simulink model "cooperative_observer"  (R2024b)
settings: Solver=VariableStepAuto  StartTime=0.0  StopTime=T_sim  RelTol=1e-3
undefined symbols (not defined in the file): A0, Adj, B, C, c, D, F_c, G, K, L0, noise_level, noise_sample_time, x0_0, x0_1, x0_2, x0_3, x0_4, x0_5, x0_6, x0_hat
libraries: simulink x7
settings Model: Creator=fvero  LastModifiedBy=fvero

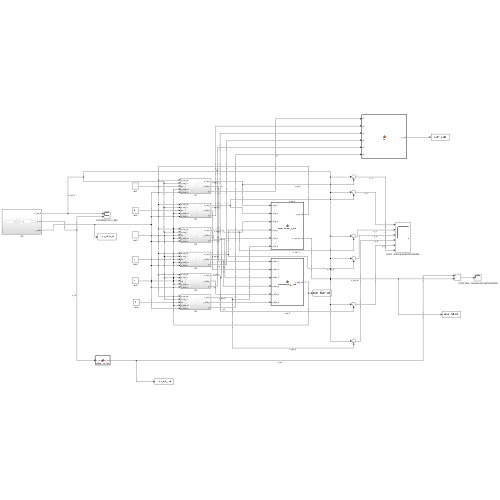
[thumbnail: Simulink's stored preview of the top-level diagram]
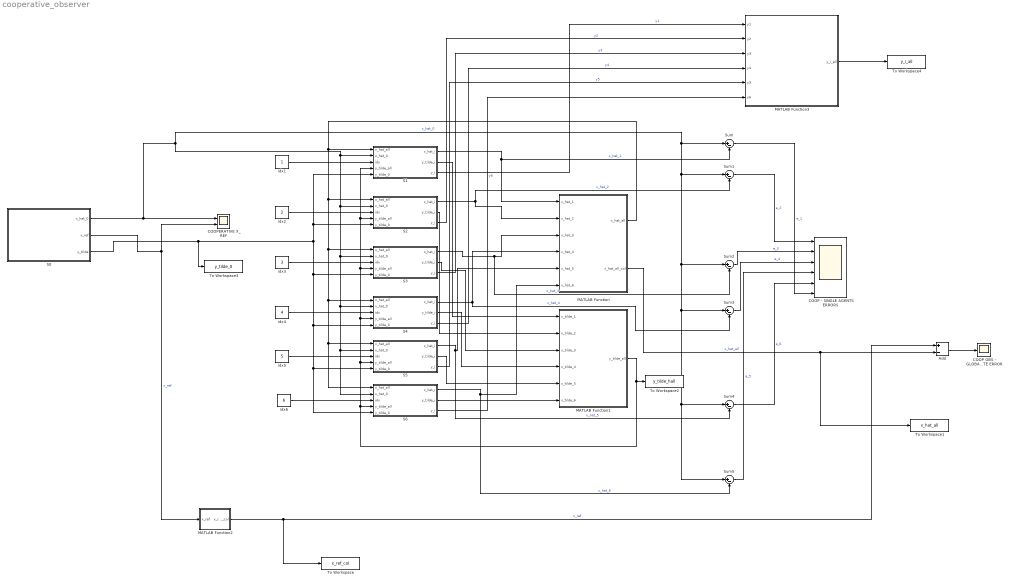
== system cooperative_observer ==
  Add : Sum  Inputs=+-
  "COOP - SINGLE AGENTS ERRORS " : Scope  NumInputPorts=6
  COOP OBS - GLOBAL ESTIMATE ERROR : Scope
  COOPERATIVE X_REF : Scope  NumInputPorts=2
  MATLAB Function : MATLAB Function  TreatAsAtomicUnit=on
  MATLAB Function1 : MATLAB Function  TreatAsAtomicUnit=on
  MATLAB Function2 : MATLAB Function  TreatAsAtomicUnit=on
  MATLAB Function3 : MATLAB Function  TreatAsAtomicUnit=on
  S0 : Subsystem
  S1 : Subsystem
  S2 : Subsystem
  S3 : Subsystem
  S4 : Subsystem
  S5 : Subsystem
  S6 : Subsystem
  Sum{,1..5} (6 alike) : Sum  Inputs=|+-
  To Workspace : ToWorkspace  VariableName=x_ref_col  SaveFormat=Timeseries  SampleTime=-1
  To Workspace1 : ToWorkspace  VariableName=x_hat_all  SaveFormat=Timeseries  SampleTime=-1
  To Workspace2 : ToWorkspace  VariableName=y_tilde_hall  SaveFormat=Timeseries  SampleTime=-1
  To Workspace3 : ToWorkspace  VariableName=y_tilde_0  SaveFormat=Timeseries  SampleTime=-1
  To Workspace4 : ToWorkspace  VariableName=y_i_all  SaveFormat=Timeseries  SampleTime=-1
  idx1 : Constant
  idx2 : Constant  Value=2
  idx3 : Constant  Value=3
  idx4 : Constant  Value=4
  idx5 : Constant  Value=5
  idx6 : Constant  Value=6
  wires:
  MATLAB Function/1(x_hat_all) -> S2/1(x_hat_all), S3/1(x_hat_all), S6/1(x_hat_all), S5/1(x_hat_all), S4/1(x_hat_all), S1/1(x_hat_all)
  idx1/1 -> S1/3(idx)
  idx2/1 -> S2/3(idx)
  idx3/1 -> S3/3(idx)
  idx4/1 -> S4/3(idx)
  idx6/1 -> S6/3(idx)
  idx5/1 -> S5/3(idx)
  S0/1(x_hat_0) -> S2/2(x_hat_0), S3/2(x_hat_0), S6/2(x_hat_0), S5/2(x_hat_0), S4/2(x_hat_0), S1/2(x_hat_0), Sum4/1, Sum5/1, Sum3/1, Sum2/1, Sum1/1, Sum/1, COOPERATIVE X_REF/1  "x_hat_0"
  S1/1(x_hat_i) -> Sum/2, MATLAB Function/1(x_hat_1)  "x_hat_1"
  S2/1(x_hat_i) -> MATLAB Function/2(x_hat_2), Sum1/2  "x_hat_2"
  S3/1(x_hat_i) -> Sum2/2, MATLAB Function/3(x_hat_3)  "x_hat_3"
  S4/1(x_hat_i) -> MATLAB Function/4(x_hat_4), Sum3/2  "x_hat_4"
  S5/1(x_hat_i) -> Sum4/2, MATLAB Function/5(x_hat_5)  "x_hat_5"
  S6/1(x_hat_i) -> Sum5/2, MATLAB Function/6(x_hat_6)  "x_hat_6"
  S1/2(y_tilde_i) -> MATLAB Function1/1(x_tilde_1)
  S2/2(y_tilde_i) -> MATLAB Function1/2(x_tilde_2)
  S3/2(y_tilde_i) -> MATLAB Function1/3(x_tilde_3)
  S4/2(y_tilde_i) -> MATLAB Function1/4(x_tilde_4)
  S5/2(y_tilde_i) -> MATLAB Function1/5(x_tilde_5)
  S6/2(y_tilde_i) -> MATLAB Function1/6(x_tilde_6)
  MATLAB Function1/1(y_tilde_all) -> To Workspace2/1, S6/4(y_tilde_all), S5/4(y_tilde_all), S4/4(y_tilde_all), S3/4(y_tilde_all), S2/4(y_tilde_all), S1/4(y_tilde_all)
  S0/3(y_tilde) -> To Workspace3/1, S2/5(y_tilde_0), S1/5(y_tilde_0), S3/5(y_tilde_0), S6/5(y_tilde_0), S5/5(y_tilde_0), S4/5(y_tilde_0)
  MATLAB Function/2(x_hat_all_col) -> To Workspace1/1, Add/2  "x_hat_all"
  S0/2(x_ref) -> MATLAB Function2/1(x_ref), COOPERATIVE X_REF/2  "x_ref"
  MATLAB Function2/1(x_ref_col) -> To Workspace/1, Add/1  "x_ref"
  Add/1 -> COOP OBS - GLOBAL ESTIMATE ERROR/1
  Sum/1 -> "COOP - SINGLE AGENTS ERRORS "/6  "e_1"
  Sum1/1 -> "COOP - SINGLE AGENTS ERRORS "/1  "e_2"
  Sum2/1 -> "COOP - SINGLE AGENTS ERRORS "/2  "e_3"
  Sum3/1 -> "COOP - SINGLE AGENTS ERRORS "/3  "e_4"
  Sum4/1 -> "COOP - SINGLE AGENTS ERRORS "/5  "e_6"
  Sum5/1 -> "COOP - SINGLE AGENTS ERRORS "/4  "e_5"
  S1/3(y_i) -> MATLAB Function3/1(y1)  "y1"
  S2/3(y_i) -> MATLAB Function3/2(y2)  "y2"
  S3/3(y_i) -> MATLAB Function3/3(y3)  "y3"
  S4/3(y_i) -> MATLAB Function3/4(y4)  "y4"
  S5/3(y_i) -> MATLAB Function3/5(y5)  "y5"
  S6/3(y_i) -> MATLAB Function3/6(y6)  "y6"
  MATLAB Function3/1(y_i_all) -> To Workspace4/1

== system cooperative_observer/S0 ==
  Leader Observer : Subsystem
  Subsystem : Subsystem
  To Workspace : ToWorkspace  VariableName=y_ref  SaveFormat=Timeseries  SampleTime=-1
  x_hat_0 : Outport
  x_ref : Outport  Port=2
  y_tilde : Outport  Port=3
  wires:
  Subsystem/1(y_ref) -> To Workspace/1, Leader Observer/1(y)
  Leader Observer/1(x_hat_0) -> x_hat_0/1
  Subsystem/2(x_ref) -> x_ref/1
  Leader Observer/2(y_tilde) -> y_tilde/1

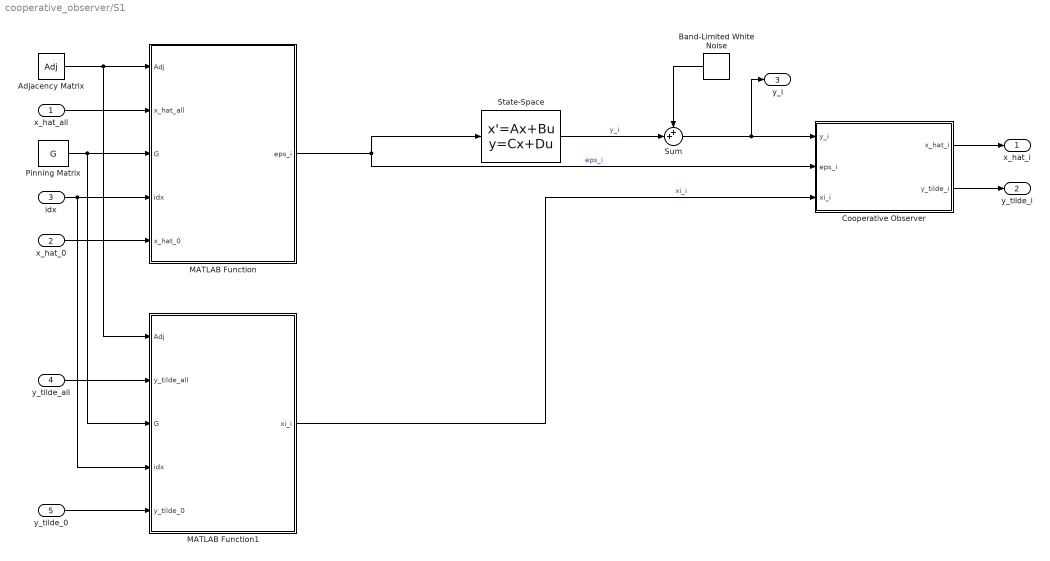
== system cooperative_observer/S1 ==
  x_hat_all : Inport
  x_hat_0 : Inport  Port=2
  idx : Inport  Port=3
  y_tilde_all : Inport  Port=4
  y_tilde_0 : Inport  Port=5
  "Adjacency Matrix " : Constant  Value=Adj
  Band-Limited White Noise : simulink/Sources/Band-Limited White Noise  Cov=[noise_level]  Ts=noise_sample_time  seed=[42]
  Cooperative Observer : Subsystem
  MATLAB Function : MATLAB Function  TreatAsAtomicUnit=on
  MATLAB Function1 : MATLAB Function  TreatAsAtomicUnit=on
  Pinning Matrix : Constant  Value=G
  State-Space : StateSpace  A=A0  B=c*B*K  C=C  D=D  InitialCondition=x0_1
  Sum : Sum  Inputs=++|
  x_hat_i : Outport
  y_tilde_i : Outport  Port=2
  y_i : Outport  Port=3
  wires:
  MATLAB Function/1(eps_i) -> State-Space/1, Cooperative Observer/2(eps_i)  "eps_i"
  x_hat_all/1 -> MATLAB Function/2(x_hat_all)
  x_hat_0/1 -> MATLAB Function/5(x_hat_0)
  Pinning Matrix/1 -> MATLAB Function1/3(G), MATLAB Function/3(G)
  "Adjacency Matrix "/1 -> MATLAB Function1/1(Adj), MATLAB Function/1(Adj)
  idx/1 -> MATLAB Function1/4(idx), MATLAB Function/4(idx)
  Cooperative Observer/1(x_hat_i) -> x_hat_i/1
  Cooperative Observer/2(y_tilde_i) -> y_tilde_i/1
  y_tilde_all/1 -> MATLAB Function1/2(y_tilde_all)
  y_tilde_0/1 -> MATLAB Function1/5(y_tilde_0)
  MATLAB Function1/1(xi_i) -> Cooperative Observer/3(xi_i)  "xi_i"
  Band-Limited White Noise/1 -> Sum/1
  State-Space/1 -> Sum/2  "y_i"
  Sum/1 -> y_i/1, Cooperative Observer/1(y_i)

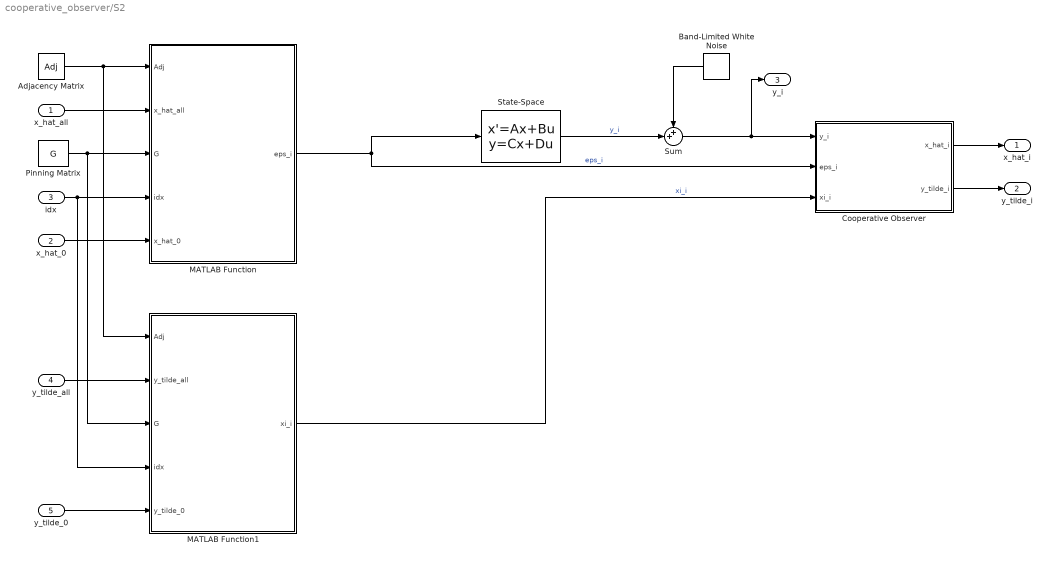
== system cooperative_observer/S2 ==
  x_hat_all : Inport
  x_hat_0 : Inport  Port=2
  idx : Inport  Port=3
  y_tilde_all : Inport  Port=4
  y_tilde_0 : Inport  Port=5
  "Adjacency Matrix " : Constant  Value=Adj
  Band-Limited White Noise : simulink/Sources/Band-Limited White Noise  Cov=[noise_level]  Ts=noise_sample_time  seed=[42]
  Cooperative Observer : Subsystem
  MATLAB Function : MATLAB Function  TreatAsAtomicUnit=on
  MATLAB Function1 : MATLAB Function  TreatAsAtomicUnit=on
  Pinning Matrix : Constant  Value=G
  State-Space : StateSpace  A=A0  B=c*B*K  C=C  D=D  InitialCondition=x0_2
  Sum : Sum  Inputs=++|
  x_hat_i : Outport
  y_tilde_i : Outport  Port=2
  y_i : Outport  Port=3
  wires:
  MATLAB Function/1(eps_i) -> State-Space/1, Cooperative Observer/2(eps_i)  "eps_i"
  x_hat_all/1 -> MATLAB Function/2(x_hat_all)
  x_hat_0/1 -> MATLAB Function/5(x_hat_0)
  Pinning Matrix/1 -> MATLAB Function1/3(G), MATLAB Function/3(G)
  "Adjacency Matrix "/1 -> MATLAB Function1/1(Adj), MATLAB Function/1(Adj)
  idx/1 -> MATLAB Function1/4(idx), MATLAB Function/4(idx)
  Cooperative Observer/1(x_hat_i) -> x_hat_i/1
  Cooperative Observer/2(y_tilde_i) -> y_tilde_i/1
  y_tilde_all/1 -> MATLAB Function1/2(y_tilde_all)
  y_tilde_0/1 -> MATLAB Function1/5(y_tilde_0)
  MATLAB Function1/1(xi_i) -> Cooperative Observer/3(xi_i)  "xi_i"
  Band-Limited White Noise/1 -> Sum/1
  State-Space/1 -> Sum/2  "y_i"
  Sum/1 -> y_i/1, Cooperative Observer/1(y_i)

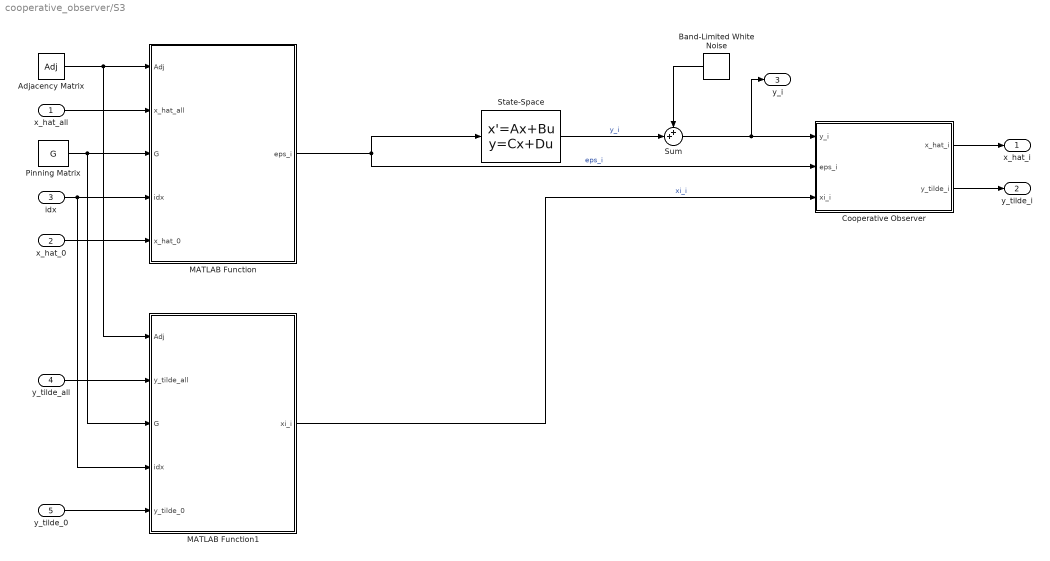
== system cooperative_observer/S3 ==
  x_hat_all : Inport
  x_hat_0 : Inport  Port=2
  idx : Inport  Port=3
  y_tilde_all : Inport  Port=4
  y_tilde_0 : Inport  Port=5
  "Adjacency Matrix " : Constant  Value=Adj
  Band-Limited White Noise : simulink/Sources/Band-Limited White Noise  Cov=[noise_level]  Ts=noise_sample_time  seed=[42]
  Cooperative Observer : Subsystem
  MATLAB Function : MATLAB Function  TreatAsAtomicUnit=on
  MATLAB Function1 : MATLAB Function  TreatAsAtomicUnit=on
  Pinning Matrix : Constant  Value=G
  State-Space : StateSpace  A=A0  B=c*B*K  C=C  D=D  InitialCondition=x0_3
  Sum : Sum  Inputs=++|
  x_hat_i : Outport
  y_tilde_i : Outport  Port=2
  y_i : Outport  Port=3
  wires:
  MATLAB Function/1(eps_i) -> State-Space/1, Cooperative Observer/2(eps_i)  "eps_i"
  x_hat_all/1 -> MATLAB Function/2(x_hat_all)
  x_hat_0/1 -> MATLAB Function/5(x_hat_0)
  Pinning Matrix/1 -> MATLAB Function1/3(G), MATLAB Function/3(G)
  "Adjacency Matrix "/1 -> MATLAB Function1/1(Adj), MATLAB Function/1(Adj)
  idx/1 -> MATLAB Function1/4(idx), MATLAB Function/4(idx)
  Cooperative Observer/1(x_hat_i) -> x_hat_i/1
  Cooperative Observer/2(y_tilde_i) -> y_tilde_i/1
  y_tilde_all/1 -> MATLAB Function1/2(y_tilde_all)
  y_tilde_0/1 -> MATLAB Function1/5(y_tilde_0)
  MATLAB Function1/1(xi_i) -> Cooperative Observer/3(xi_i)  "xi_i"
  Band-Limited White Noise/1 -> Sum/1
  State-Space/1 -> Sum/2  "y_i"
  Sum/1 -> y_i/1, Cooperative Observer/1(y_i)

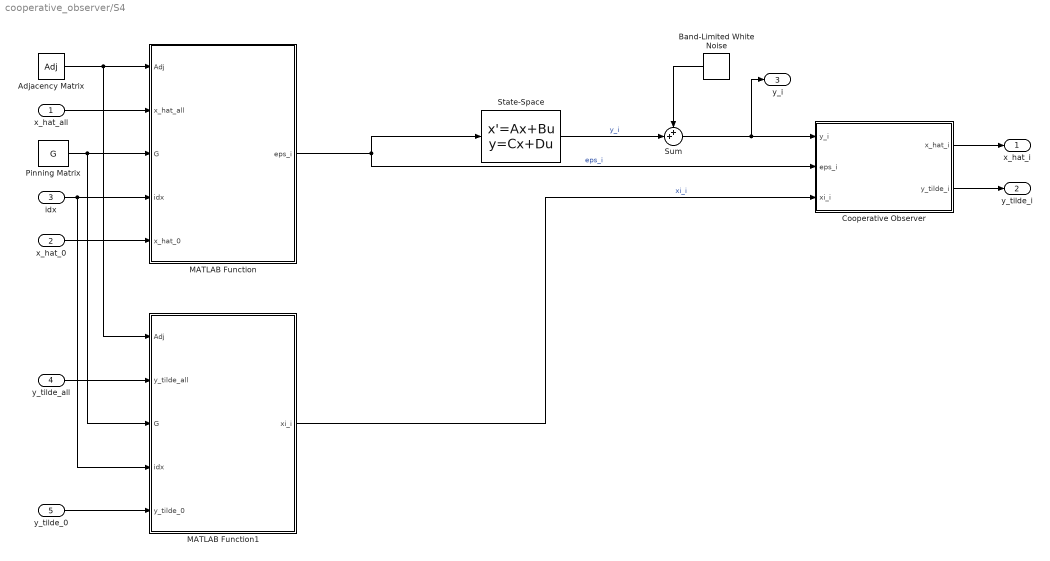
== system cooperative_observer/S4 ==
  x_hat_all : Inport
  x_hat_0 : Inport  Port=2
  idx : Inport  Port=3
  y_tilde_all : Inport  Port=4
  y_tilde_0 : Inport  Port=5
  "Adjacency Matrix " : Constant  Value=Adj
  Band-Limited White Noise : simulink/Sources/Band-Limited White Noise  Cov=[noise_level]  Ts=noise_sample_time  seed=[42]
  Cooperative Observer : Subsystem
  MATLAB Function : MATLAB Function  TreatAsAtomicUnit=on
  MATLAB Function1 : MATLAB Function  TreatAsAtomicUnit=on
  Pinning Matrix : Constant  Value=G
  State-Space : StateSpace  A=A0  B=c*B*K  C=C  D=D  InitialCondition=x0_4
  Sum : Sum  Inputs=++|
  x_hat_i : Outport
  y_tilde_i : Outport  Port=2
  y_i : Outport  Port=3
  wires:
  MATLAB Function/1(eps_i) -> State-Space/1, Cooperative Observer/2(eps_i)  "eps_i"
  x_hat_all/1 -> MATLAB Function/2(x_hat_all)
  x_hat_0/1 -> MATLAB Function/5(x_hat_0)
  Pinning Matrix/1 -> MATLAB Function1/3(G), MATLAB Function/3(G)
  "Adjacency Matrix "/1 -> MATLAB Function1/1(Adj), MATLAB Function/1(Adj)
  idx/1 -> MATLAB Function1/4(idx), MATLAB Function/4(idx)
  Cooperative Observer/1(x_hat_i) -> x_hat_i/1
  Cooperative Observer/2(y_tilde_i) -> y_tilde_i/1
  y_tilde_all/1 -> MATLAB Function1/2(y_tilde_all)
  y_tilde_0/1 -> MATLAB Function1/5(y_tilde_0)
  MATLAB Function1/1(xi_i) -> Cooperative Observer/3(xi_i)  "xi_i"
  Band-Limited White Noise/1 -> Sum/1
  State-Space/1 -> Sum/2  "y_i"
  Sum/1 -> y_i/1, Cooperative Observer/1(y_i)

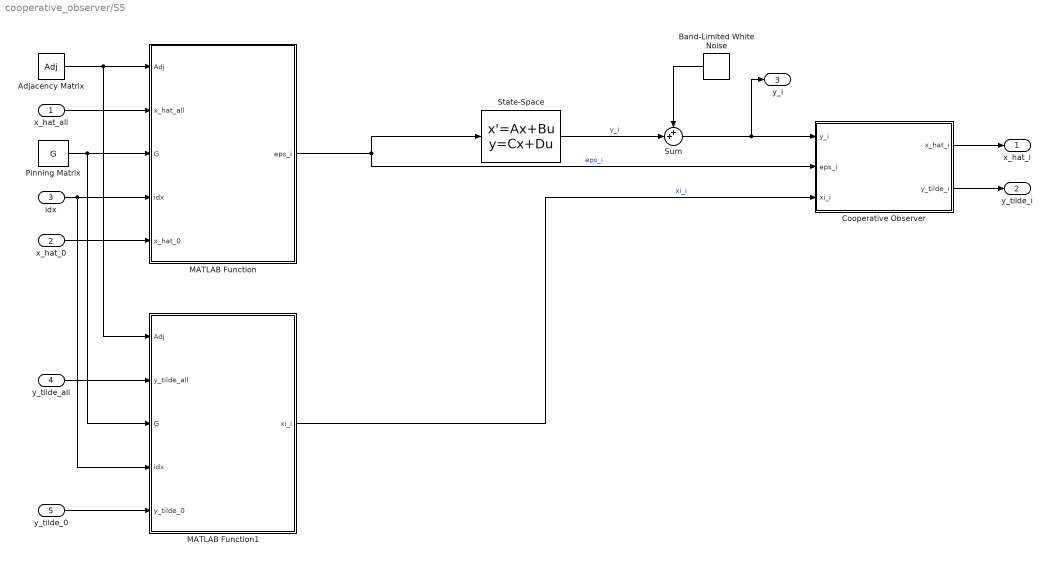
== system cooperative_observer/S5 ==
  x_hat_all : Inport
  x_hat_0 : Inport  Port=2
  idx : Inport  Port=3
  y_tilde_all : Inport  Port=4
  y_tilde_0 : Inport  Port=5
  "Adjacency Matrix " : Constant  Value=Adj
  Band-Limited White Noise : simulink/Sources/Band-Limited White Noise  Cov=[noise_level]  Ts=noise_sample_time  seed=[42]
  Cooperative Observer : Subsystem
  MATLAB Function : MATLAB Function  TreatAsAtomicUnit=on
  MATLAB Function1 : MATLAB Function  TreatAsAtomicUnit=on
  Pinning Matrix : Constant  Value=G
  State-Space : StateSpace  A=A0  B=c*B*K  C=C  D=D  InitialCondition=x0_5
  Sum : Sum  Inputs=++|
  x_hat_i : Outport
  y_tilde_i : Outport  Port=2
  y_i : Outport  Port=3
  wires:
  MATLAB Function/1(eps_i) -> State-Space/1, Cooperative Observer/2(eps_i)  "eps_i"
  x_hat_all/1 -> MATLAB Function/2(x_hat_all)
  x_hat_0/1 -> MATLAB Function/5(x_hat_0)
  Pinning Matrix/1 -> MATLAB Function1/3(G), MATLAB Function/3(G)
  "Adjacency Matrix "/1 -> MATLAB Function1/1(Adj), MATLAB Function/1(Adj)
  idx/1 -> MATLAB Function1/4(idx), MATLAB Function/4(idx)
  Cooperative Observer/1(x_hat_i) -> x_hat_i/1
  Cooperative Observer/2(y_tilde_i) -> y_tilde_i/1
  y_tilde_all/1 -> MATLAB Function1/2(y_tilde_all)
  y_tilde_0/1 -> MATLAB Function1/5(y_tilde_0)
  MATLAB Function1/1(xi_i) -> Cooperative Observer/3(xi_i)  "xi_i"
  Band-Limited White Noise/1 -> Sum/1
  State-Space/1 -> Sum/2  "y_i"
  Sum/1 -> y_i/1, Cooperative Observer/1(y_i)

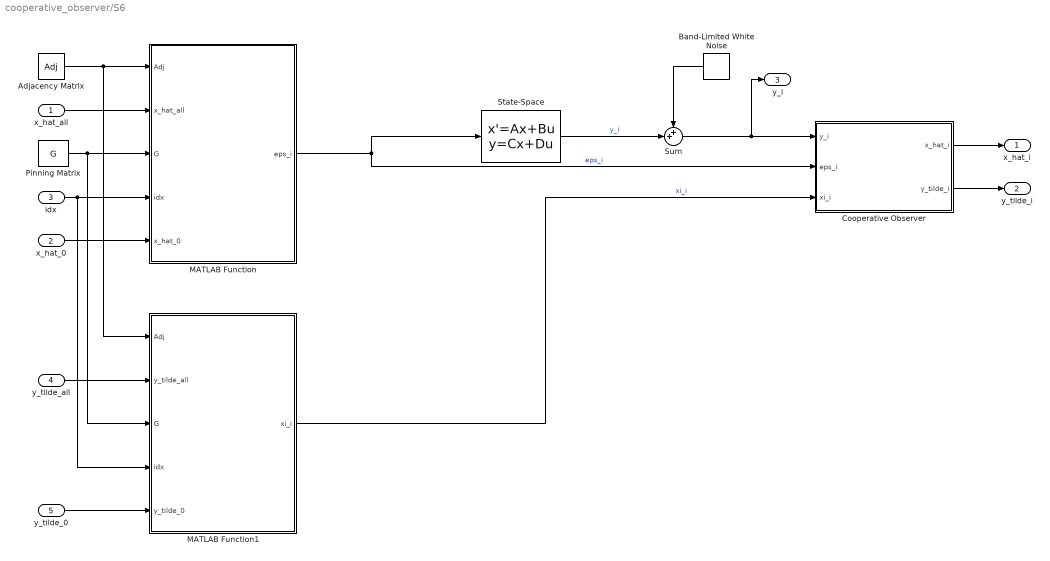
== system cooperative_observer/S6 ==
  x_hat_all : Inport
  x_hat_0 : Inport  Port=2
  idx : Inport  Port=3
  y_tilde_all : Inport  Port=4
  y_tilde_0 : Inport  Port=5
  "Adjacency Matrix " : Constant  Value=Adj
  Band-Limited White Noise : simulink/Sources/Band-Limited White Noise  Cov=[noise_level]  Ts=noise_sample_time  seed=[42]
  Cooperative Observer : Subsystem
  MATLAB Function : MATLAB Function  TreatAsAtomicUnit=on
  MATLAB Function1 : MATLAB Function  TreatAsAtomicUnit=on
  Pinning Matrix : Constant  Value=G
  State-Space : StateSpace  A=A0  B=c*B*K  C=C  D=D  InitialCondition=x0_6
  Sum : Sum  Inputs=++|
  x_hat_i : Outport
  y_tilde_i : Outport  Port=2
  y_i : Outport  Port=3
  wires:
  MATLAB Function/1(eps_i) -> State-Space/1, Cooperative Observer/2(eps_i)  "eps_i"
  x_hat_all/1 -> MATLAB Function/2(x_hat_all)
  x_hat_0/1 -> MATLAB Function/5(x_hat_0)
  Pinning Matrix/1 -> MATLAB Function1/3(G), MATLAB Function/3(G)
  "Adjacency Matrix "/1 -> MATLAB Function1/1(Adj), MATLAB Function/1(Adj)
  idx/1 -> MATLAB Function1/4(idx), MATLAB Function/4(idx)
  Cooperative Observer/1(x_hat_i) -> x_hat_i/1
  Cooperative Observer/2(y_tilde_i) -> y_tilde_i/1
  y_tilde_all/1 -> MATLAB Function1/2(y_tilde_all)
  y_tilde_0/1 -> MATLAB Function1/5(y_tilde_0)
  MATLAB Function1/1(xi_i) -> Cooperative Observer/3(xi_i)  "xi_i"
  Band-Limited White Noise/1 -> Sum/1
  State-Space/1 -> Sum/2  "y_i"
  Sum/1 -> y_i/1, Cooperative Observer/1(y_i)

== system cooperative_observer/S0/Leader Observer ==
  y : Inport
  Add : Sum
  Add1 : Sum  Inputs=+-
  Band-Limited White Noise : simulink/Sources/Band-Limited White Noise  Cov=noise_level  Ts=noise_sample_time  seed=[42]
  Gain1 : Gain  Gain=A0  Multiplication=Matrix(K*u)
  Gain2 : Gain  Gain=C  Multiplication=Matrix(K*u)
  Gain3 : Gain  Gain=c*L0  Multiplication=Matrix(K*u)
  Integrator : Integrator  InitialCondition=[0, 0]'
  Sum : Sum  Inputs=|++
  x_hat_0 : Outport
  y_tilde : Outport  Port=2
  wires:
  Add/1 -> Integrator/1  "x_hat_dot"
  Integrator/1 -> x_hat_0/1, Gain2/1, Gain1/1  "x_hat"
  Gain2/1 -> Add1/2  "y_hat"
  Gain1/1 -> Add/2
  Add1/1 -> y_tilde/1, Gain3/1  "y_tilde"
  Gain3/1 -> Add/1
  Band-Limited White Noise/1 -> Sum/2
  y/1 -> Sum/1
  Sum/1 -> Add1/1

== system cooperative_observer/S0/Subsystem ==
  Gain : Gain  Gain=C  Multiplication=Matrix(K*u)
  Gain1 : Gain  Gain=A0  Multiplication=Matrix(K*u)
  Integrator : Integrator  InitialCondition=x0_0
  y_ref : Outport
  x_ref : Outport  Port=2
  wires:
  Gain1/1 -> Integrator/1
  Integrator/1 -> Gain1/1, Gain/1, x_ref/1
  Gain/1 -> y_ref/1

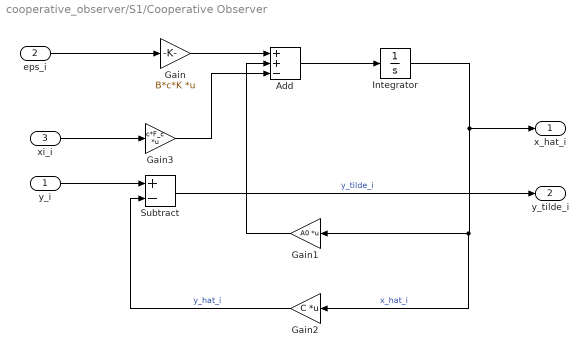
== system cooperative_observer/S1/Cooperative Observer ==
  y_i : Inport
  eps_i : Inport  Port=2
  xi_i : Inport  Port=3
  Add : Sum  Inputs=++-
  Gain : Gain  Gain=B*c*K  Multiplication=Matrix(K*u)
  Gain1 : Gain  Gain=A0  Multiplication=Matrix(K*u)
  Gain2 : Gain  Gain=C  Multiplication=Matrix(K*u)
  Gain3 : Gain  Gain=c*F_c  Multiplication=Matrix(K*u)
  Integrator : Integrator  InitialCondition=x0_hat
  Subtract : Sum  Inputs=+-
  x_hat_i : Outport
  y_tilde_i : Outport  Port=2
  wires:
  eps_i/1 -> Gain/1
  Integrator/1 -> Gain2/1, Gain1/1, x_hat_i/1  "x_hat_i"
  y_i/1 -> Subtract/1
  Gain2/1 -> Subtract/2  "y_hat_i"
  Subtract/1 -> y_tilde_i/1  "y_tilde_i"
  Gain/1 -> Add/1
  Gain3/1 -> Add/3
  Gain1/1 -> Add/2
  Add/1 -> Integrator/1
  xi_i/1 -> Gain3/1

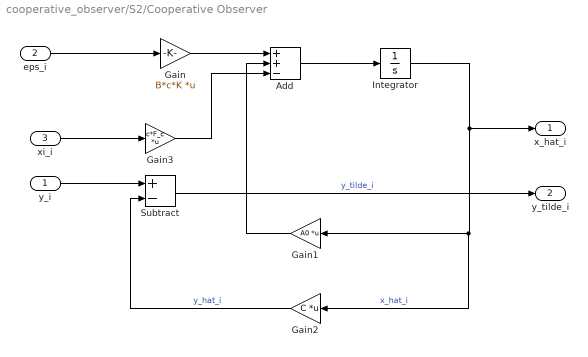
== system cooperative_observer/S2/Cooperative Observer ==
  y_i : Inport
  eps_i : Inport  Port=2
  xi_i : Inport  Port=3
  Add : Sum  Inputs=++-
  Gain : Gain  Gain=B*c*K  Multiplication=Matrix(K*u)
  Gain1 : Gain  Gain=A0  Multiplication=Matrix(K*u)
  Gain2 : Gain  Gain=C  Multiplication=Matrix(K*u)
  Gain3 : Gain  Gain=c*F_c  Multiplication=Matrix(K*u)
  Integrator : Integrator  InitialCondition=x0_hat
  Subtract : Sum  Inputs=+-
  x_hat_i : Outport
  y_tilde_i : Outport  Port=2
  wires:
  eps_i/1 -> Gain/1
  Integrator/1 -> Gain2/1, Gain1/1, x_hat_i/1  "x_hat_i"
  y_i/1 -> Subtract/1
  Gain2/1 -> Subtract/2  "y_hat_i"
  Subtract/1 -> y_tilde_i/1  "y_tilde_i"
  Gain/1 -> Add/1
  Gain3/1 -> Add/3
  Gain1/1 -> Add/2
  Add/1 -> Integrator/1
  xi_i/1 -> Gain3/1

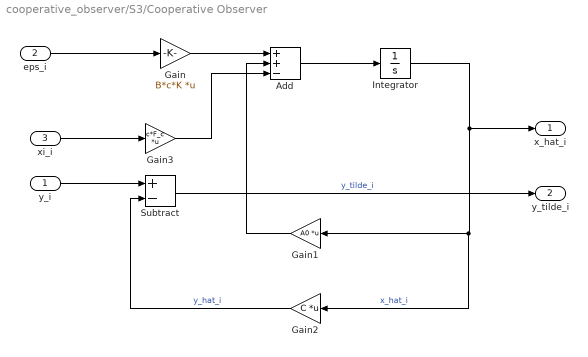
== system cooperative_observer/S3/Cooperative Observer ==
  y_i : Inport
  eps_i : Inport  Port=2
  xi_i : Inport  Port=3
  Add : Sum  Inputs=++-
  Gain : Gain  Gain=B*c*K  Multiplication=Matrix(K*u)
  Gain1 : Gain  Gain=A0  Multiplication=Matrix(K*u)
  Gain2 : Gain  Gain=C  Multiplication=Matrix(K*u)
  Gain3 : Gain  Gain=c*F_c  Multiplication=Matrix(K*u)
  Integrator : Integrator  InitialCondition=x0_hat
  Subtract : Sum  Inputs=+-
  x_hat_i : Outport
  y_tilde_i : Outport  Port=2
  wires:
  eps_i/1 -> Gain/1
  Integrator/1 -> Gain2/1, Gain1/1, x_hat_i/1  "x_hat_i"
  y_i/1 -> Subtract/1
  Gain2/1 -> Subtract/2  "y_hat_i"
  Subtract/1 -> y_tilde_i/1  "y_tilde_i"
  Gain/1 -> Add/1
  Gain3/1 -> Add/3
  Gain1/1 -> Add/2
  Add/1 -> Integrator/1
  xi_i/1 -> Gain3/1

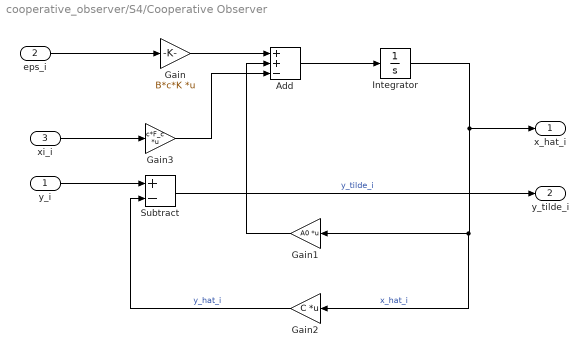
== system cooperative_observer/S4/Cooperative Observer ==
  y_i : Inport
  eps_i : Inport  Port=2
  xi_i : Inport  Port=3
  Add : Sum  Inputs=++-
  Gain : Gain  Gain=B*c*K  Multiplication=Matrix(K*u)
  Gain1 : Gain  Gain=A0  Multiplication=Matrix(K*u)
  Gain2 : Gain  Gain=C  Multiplication=Matrix(K*u)
  Gain3 : Gain  Gain=c*F_c  Multiplication=Matrix(K*u)
  Integrator : Integrator  InitialCondition=x0_hat
  Subtract : Sum  Inputs=+-
  x_hat_i : Outport
  y_tilde_i : Outport  Port=2
  wires:
  eps_i/1 -> Gain/1
  Integrator/1 -> Gain2/1, Gain1/1, x_hat_i/1  "x_hat_i"
  y_i/1 -> Subtract/1
  Gain2/1 -> Subtract/2  "y_hat_i"
  Subtract/1 -> y_tilde_i/1  "y_tilde_i"
  Gain/1 -> Add/1
  Gain3/1 -> Add/3
  Gain1/1 -> Add/2
  Add/1 -> Integrator/1
  xi_i/1 -> Gain3/1

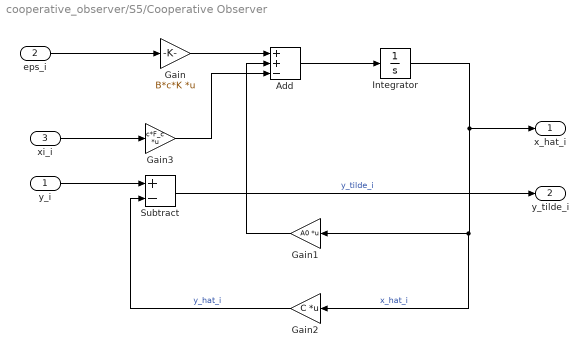
== system cooperative_observer/S5/Cooperative Observer ==
  y_i : Inport
  eps_i : Inport  Port=2
  xi_i : Inport  Port=3
  Add : Sum  Inputs=++-
  Gain : Gain  Gain=B*c*K  Multiplication=Matrix(K*u)
  Gain1 : Gain  Gain=A0  Multiplication=Matrix(K*u)
  Gain2 : Gain  Gain=C  Multiplication=Matrix(K*u)
  Gain3 : Gain  Gain=c*F_c  Multiplication=Matrix(K*u)
  Integrator : Integrator  InitialCondition=x0_hat
  Subtract : Sum  Inputs=+-
  x_hat_i : Outport
  y_tilde_i : Outport  Port=2
  wires:
  eps_i/1 -> Gain/1
  Integrator/1 -> Gain2/1, Gain1/1, x_hat_i/1  "x_hat_i"
  y_i/1 -> Subtract/1
  Gain2/1 -> Subtract/2  "y_hat_i"
  Subtract/1 -> y_tilde_i/1  "y_tilde_i"
  Gain/1 -> Add/1
  Gain3/1 -> Add/3
  Gain1/1 -> Add/2
  Add/1 -> Integrator/1
  xi_i/1 -> Gain3/1

== system cooperative_observer/S6/Cooperative Observer ==
  y_i : Inport
  eps_i : Inport  Port=2
  xi_i : Inport  Port=3
  Add : Sum  Inputs=++-
  Gain : Gain  Gain=B*c*K  Multiplication=Matrix(K*u)
  Gain1 : Gain  Gain=A0  Multiplication=Matrix(K*u)
  Gain2 : Gain  Gain=C  Multiplication=Matrix(K*u)
  Gain3 : Gain  Gain=c*F_c  Multiplication=Matrix(K*u)
  Integrator : Integrator  InitialCondition=x0_hat
  Subtract : Sum  Inputs=+-
  x_hat_i : Outport
  y_tilde_i : Outport  Port=2
  wires:
  eps_i/1 -> Gain/1
  Integrator/1 -> Gain2/1, Gain1/1, x_hat_i/1  "x_hat_i"
  y_i/1 -> Subtract/1
  Gain2/1 -> Subtract/2  "y_hat_i"
  Subtract/1 -> y_tilde_i/1  "y_tilde_i"
  Gain/1 -> Add/1
  Gain3/1 -> Add/3
  Gain1/1 -> Add/2
  Add/1 -> Integrator/1
  xi_i/1 -> Gain3/1

== matlab function cooperative_observer/S4/MATLAB Function1 ==
  data: Adj input; xi_i output; y_tilde_all input; G input; idx input; y_tilde_0 input
function xi_i = compute_xi(Adj, y_tilde_all, G, idx, y_tilde_0)

Adj_i = Adj(idx, :);
g_i = G(idx, idx);

y_tilde_i = y_tilde_all(idx); 

diff = g_i * (y_tilde_0 - y_tilde_i); 

xi_i = 0; 

for j = 1:6
    xi_i = xi_i + Adj_i(j)*(y_tilde_all(j) - y_tilde_i); 
end 

xi_i = xi_i + diff;

end

== matlab function cooperative_observer/S5/MATLAB Function ==
  data: Adj input; eps_i output; x_hat_all input; G input; idx input; x_hat_0 input
function eps_i = compute_eps(Adj, x_hat_all, G, idx, x_hat_0)

Adj_i = Adj(idx, :);
g_i = G(idx, idx);

x_hat_i = x_hat_all(idx, :)'; %2*1

diff = g_i * (x_hat_0 - x_hat_i); 

eps_i = zeros(size(x_hat_i)); 

for j = 1:6
    eps_i = eps_i + Adj_i(j)*(x_hat_all(j,:)' - x_hat_i); 
end 

eps_i = eps_i + diff; 

end

== matlab function cooperative_observer/S5/MATLAB Function1 ==
  data: Adj input; xi_i output; y_tilde_all input; G input; idx input; y_tilde_0 input
function xi_i = compute_xi(Adj, y_tilde_all, G, idx, y_tilde_0)

Adj_i = Adj(idx, :);
g_i = G(idx, idx);

y_tilde_i = y_tilde_all(idx); 

diff = g_i * (y_tilde_0 - y_tilde_i); 

xi_i = 0; 

for j = 1:6
    xi_i = xi_i + Adj_i(j)*(y_tilde_all(j) - y_tilde_i); 
end 

xi_i = xi_i + diff;

end

== matlab function cooperative_observer/MATLAB Function1 ==
  data: x_tilde_1 input; y_tilde_all output; x_tilde_2 input; x_tilde_3 input; x_tilde_4 input; x_tilde_5 input; x_tilde_6 input
function y_tilde_all = concatenate_y_tilde(x_tilde_1, x_tilde_2, x_tilde_3, x_tilde_4, x_tilde_5, x_tilde_6)

y_tilde_all = [x_tilde_1 x_tilde_2 x_tilde_3 x_tilde_4 x_tilde_5 x_tilde_6];

end

== matlab function cooperative_observer/S6/MATLAB Function ==
  data: Adj input; eps_i output; x_hat_all input; G input; idx input; x_hat_0 input
function eps_i = compute_eps(Adj, x_hat_all, G, idx, x_hat_0)

Adj_i = Adj(idx, :);
g_i = G(idx, idx);

x_hat_i = x_hat_all(idx, :)'; %2*1

diff = g_i * (x_hat_0 - x_hat_i); 

eps_i = zeros(size(x_hat_i)); 

for j = 1:6
    eps_i = eps_i + Adj_i(j)*(x_hat_all(j,:)' - x_hat_i); 
end 

eps_i = eps_i + diff; 

end

== matlab function cooperative_observer/S6/MATLAB Function1 ==
  data: Adj input; xi_i output; y_tilde_all input; G input; idx input; y_tilde_0 input
function xi_i = compute_xi(Adj, y_tilde_all, G, idx, y_tilde_0)

Adj_i = Adj(idx, :);
g_i = G(idx, idx);

y_tilde_i = y_tilde_all(idx); 

diff = g_i * (y_tilde_0 - y_tilde_i); 

xi_i = 0; 

for j = 1:6
    xi_i = xi_i + Adj_i(j)*(y_tilde_all(j) - y_tilde_i); 
end 

xi_i = xi_i + diff;

end

== matlab function cooperative_observer/MATLAB Function2 ==
  data: x_ref input; x_ref_col output
function x_ref_col = repeat_vector(x_ref)

x_ref_col = repmat(x_ref, 6, 1);

== matlab function cooperative_observer/MATLAB Function3 ==
  data: y1 input; y_i_all output; y2 input; y3 input; y4 input; y5 input; y6 input
function y_i_all = fcn(y1,y2,y3,y4,y5,y6)

y_i_all = [y1,y2,y3,y4,y5,y6]';

== matlab function cooperative_observer/MATLAB Function ==
  data: x_hat_1 input; x_hat_all output; x_hat_2 input; x_hat_3 input; x_hat_4 input; x_hat_5 input; x_hat_6 input; x_hat_all_col output
function [x_hat_all, x_hat_all_col] = concatenate_x_hat(x_hat_1, x_hat_2, x_hat_3, x_hat_4, x_hat_5, x_hat_6)

x_hat_all = [x_hat_1'; x_hat_2'; x_hat_3'; x_hat_4'; x_hat_5'; x_hat_6'];
x_hat_all_col = [x_hat_1; x_hat_2; x_hat_3; x_hat_4; x_hat_5; x_hat_6];

end

== matlab function cooperative_observer/S1/MATLAB Function ==
  data: Adj input; eps_i output; x_hat_all input; G input; idx input; x_hat_0 input
function eps_i = compute_eps(Adj, x_hat_all, G, idx, x_hat_0)

Adj_i = Adj(idx, :);
g_i = G(idx, idx);

x_hat_i = x_hat_all(idx, :)'; %2*1

diff = g_i * (x_hat_0 - x_hat_i); 

eps_i = zeros(size(x_hat_i)); 

for j = 1:6
    eps_i = eps_i + Adj_i(j)*(x_hat_all(j,:)' - x_hat_i); 
end 

eps_i = eps_i + diff; 

end

== matlab function cooperative_observer/S1/MATLAB Function1 ==
  data: Adj input; xi_i output; y_tilde_all input; G input; idx input; y_tilde_0 input
function xi_i = compute_xi(Adj, y_tilde_all, G, idx, y_tilde_0)

Adj_i = Adj(idx, :);
g_i = G(idx, idx);

y_tilde_i = y_tilde_all(idx); 

diff = g_i * (y_tilde_0 - y_tilde_i); 

xi_i = 0; 

for j = 1:6
    xi_i = xi_i + Adj_i(j)*(y_tilde_all(j) - y_tilde_i); 
end 

xi_i = xi_i + diff;

end

== matlab function cooperative_observer/S2/MATLAB Function ==
  data: Adj input; eps_i output; x_hat_all input; G input; idx input; x_hat_0 input
function eps_i = compute_eps(Adj, x_hat_all, G, idx, x_hat_0)

Adj_i = Adj(idx, :);
g_i = G(idx, idx);

x_hat_i = x_hat_all(idx, :)'; %2*1

diff = g_i * (x_hat_0 - x_hat_i); 

eps_i = zeros(size(x_hat_i)); 

for j = 1:6
    eps_i = eps_i + Adj_i(j)*(x_hat_all(j,:)' - x_hat_i); 
end 

eps_i = eps_i + diff; 

end

== matlab function cooperative_observer/S2/MATLAB Function1 ==
  data: Adj input; xi_i output; y_tilde_all input; G input; idx input; y_tilde_0 input
function xi_i = compute_xi(Adj, y_tilde_all, G, idx, y_tilde_0)

Adj_i = Adj(idx, :);
g_i = G(idx, idx);

y_tilde_i = y_tilde_all(idx); 

diff = g_i * (y_tilde_0 - y_tilde_i); 

xi_i = 0; 

for j = 1:6
    xi_i = xi_i + Adj_i(j)*(y_tilde_all(j) - y_tilde_i); 
end 

xi_i = xi_i + diff;

end

== matlab function cooperative_observer/S3/MATLAB Function ==
  data: Adj input; eps_i output; x_hat_all input; G input; idx input; x_hat_0 input
function eps_i = compute_eps(Adj, x_hat_all, G, idx, x_hat_0)

Adj_i = Adj(idx, :);
g_i = G(idx, idx);

x_hat_i = x_hat_all(idx, :)'; %2*1

diff = g_i * (x_hat_0 - x_hat_i); 

eps_i = zeros(size(x_hat_i)); 

for j = 1:6
    eps_i = eps_i + Adj_i(j)*(x_hat_all(j,:)' - x_hat_i); 
end 

eps_i = eps_i + diff; 

end

== matlab function cooperative_observer/S3/MATLAB Function1 ==
  data: Adj input; xi_i output; y_tilde_all input; G input; idx input; y_tilde_0 input
function xi_i = compute_xi(Adj, y_tilde_all, G, idx, y_tilde_0)

Adj_i = Adj(idx, :);
g_i = G(idx, idx);

y_tilde_i = y_tilde_all(idx); 

diff = g_i * (y_tilde_0 - y_tilde_i); 

xi_i = 0; 

for j = 1:6
    xi_i = xi_i + Adj_i(j)*(y_tilde_all(j) - y_tilde_i); 
end 

xi_i = xi_i + diff;

end

== matlab function cooperative_observer/S4/MATLAB Function ==
  data: Adj input; eps_i output; x_hat_all input; G input; idx input; x_hat_0 input
function eps_i = compute_eps(Adj, x_hat_all, G, idx, x_hat_0)

Adj_i = Adj(idx, :);
g_i = G(idx, idx);

x_hat_i = x_hat_all(idx, :)'; %2*1

diff = g_i * (x_hat_0 - x_hat_i); 

eps_i = zeros(size(x_hat_i)); 

for j = 1:6
    eps_i = eps_i + Adj_i(j)*(x_hat_all(j,:)' - x_hat_i); 
end 

eps_i = eps_i + diff; 

end
